simulink model "state_reg_mdl_2021a"  (R2021a)
settings: Solver=VariableStepAuto  StartTime=0.0  StopTime=20  RelTol=1e-3
values from neighbouring files (symbols this model uses):
  K = acker(A, B, p)    [state_reg.m]
  reg_type = 1    [state_reg.m]
  sat_off = 1    [state_reg.m]
  T = 1e-3    (= 0.001)    [state_reg.m]
  umax = 1    [state_reg.m]
libraries: simulink x1
settings Model: Creator=rapaja  LastModifiedBy=Predrag
settings SolverCC: AlgebraicLoopSolver=TrustRegion
settings RTWCC: DLArmComputeVersion=20.02.1
settings ConfigComp: CovBoundaryAbsTol=1.0e-5

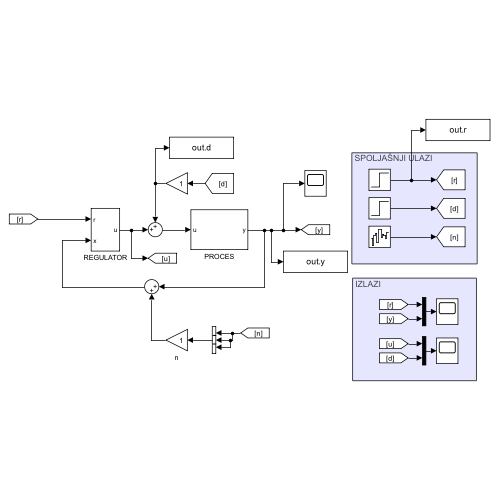
[thumbnail: Simulink's stored preview of the top-level diagram]
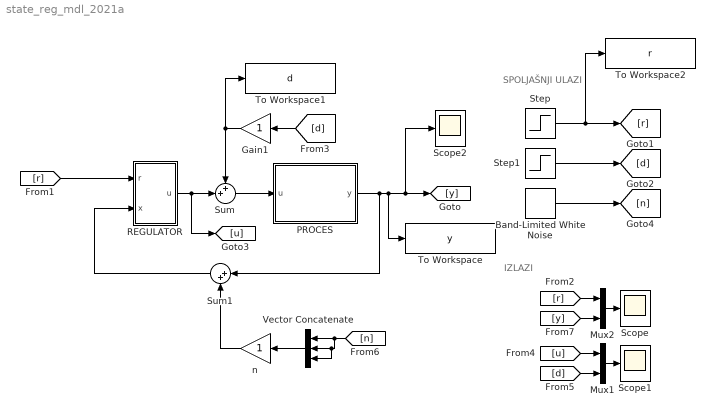
== system state_reg_mdl_2021a ==
  note: IZLAZI
  note: SPOLJAŠNJI ULAZI
  Band-Limited White Noise : simulink/Sources/Band-Limited White Noise  Cov=[0.00001]  Ts=T  seed=[23341]
  Gain1 : Gain
  Mux1 : Mux  Inputs=2
  Mux2 : Mux  Inputs=2
  PROCES : Subsystem
  REGULATOR : Subsystem
  Scope : Scope
  Scope1 : Scope
  Scope2 : Scope
  Step : Step  SampleTime=0
  Step1 : Step  Time=5  After=0  SampleTime=0
  Sum : Sum  Inputs=++|
  Sum1 : Sum  Inputs=|++
  To Workspace : ToWorkspace  VariableName=y  SampleTime=-1
  To Workspace1 : ToWorkspace  VariableName=d  SampleTime=-1
  To Workspace2 : ToWorkspace  VariableName=r  SampleTime=-1
  Vector Concatenate : Concatenate  NumInputs=3
  n : Gain
  wires:
  REGULATOR/1(u) -> [u], Sum/2
  [d] -> Gain1/1
  Band-Limited White Noise/1 -> [n]
  n/1 -> Sum1/2
  Gain1/1 -> To Workspace1/1, Sum/1
  Step1/1 -> [d]
  [r] -> Mux2/1
  [y] -> Mux2/2
  Mux2/1 -> Scope/1
  Mux1/1 -> Scope1/1
  [u] -> Mux1/1
  [d] -> Mux1/2
  PROCES/1(y) -> Sum1/1, To Workspace/1, Scope2/1, [y]
  [r] -> REGULATOR/1(r)
  Sum/1 -> PROCES/1(u)
  Sum1/1 -> REGULATOR/2(x)
  [n] -> Vector Concatenate/3, Vector Concatenate/2, Vector Concatenate/1
  Vector Concatenate/1 -> n/1
  Step/1 -> To Workspace2/1, [r]

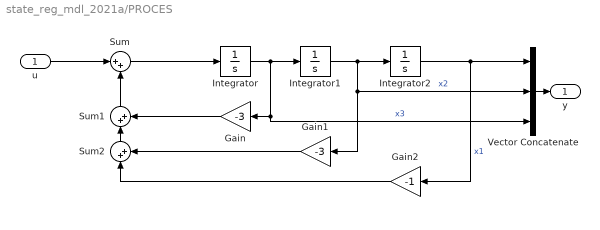
== system state_reg_mdl_2021a/PROCES ==
  u : Inport
  Gain : Gain  Gain=-3
  Gain1 : Gain  Gain=-3
  Gain2 : Gain  Gain=-1
  Integrator : Integrator
  Integrator1 : Integrator
  Integrator2 : Integrator
  Sum : Sum  Inputs=|++
  Sum1 : Sum  Inputs=|++
  Sum2 : Sum  Inputs=|++
  Vector Concatenate : Concatenate  NumInputs=3
  y : Outport
  wires:
  Vector Concatenate/1 -> y/1
  Integrator2/1 -> Gain2/1, Vector Concatenate/1  "x1"
  Integrator1/1 -> Vector Concatenate/2, Gain1/1, Integrator2/1  "x2"
  Integrator/1 -> Vector Concatenate/3, Gain/1, Integrator1/1  "x3"
  u/1 -> Sum/1
  Sum/1 -> Integrator/1
  Gain/1 -> Sum1/2
  Sum1/1 -> Sum/2
  Sum2/1 -> Sum1/1
  Gain1/1 -> Sum2/2
  Gain2/1 -> Sum2/1

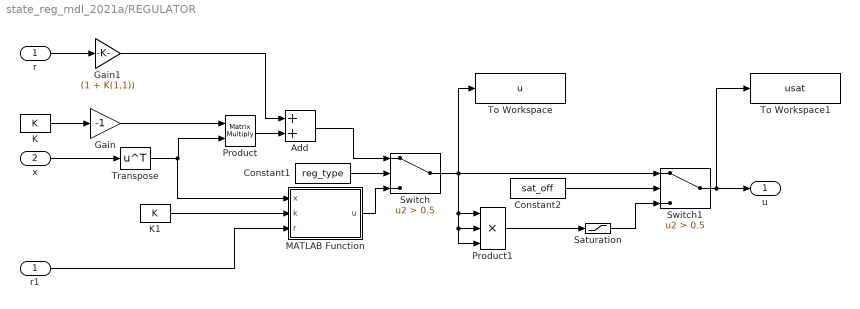
== system state_reg_mdl_2021a/REGULATOR ==
  r : Inport
  x : Inport  Port=2
  Add : Sum
  Constant1 : Constant  Value=reg_type
  Constant2 : Constant  Value=sat_off
  Gain : Gain  Gain=-1
  Gain1 : Gain  Gain=(1 + K(1,1))
  K : Constant  Value=K  VectorParams1D=off
  K1 : Constant  Value=K  VectorParams1D=off
  MATLAB Function : MATLAB Function  TreatAsAtomicUnit=on  SystemSampleTime=T
  Product : Product  Multiplication=Matrix(*)
  Product1 : Product  Inputs=3
  Saturation : Saturate  UpperLimit=umax  LowerLimit=-umax
  Switch : Switch  Criteria=u2 > Threshold  Threshold=0.5
  Switch1 : Switch  Criteria=u2 > Threshold  Threshold=0.5
  To Workspace : ToWorkspace  VariableName=u  SampleTime=-1
  To Workspace1 : ToWorkspace  VariableName=usat  SampleTime=-1
  Transpose : Math  Operator=transpose  SaturateOnIntegerOverflow=on
  r1 : InportShadow
  u : Outport
  wires:
  K/1 -> Gain/1
  r/1 -> Gain1/1
  Gain1/1 -> Add/1
  Product/1 -> Add/2
  Switch/1 -> Switch1/1, Product1/3, Product1/2, Product1/1, To Workspace/1
  MATLAB Function/1(u) -> Switch/3
  Add/1 -> Switch/1
  Constant1/1 -> Switch/2
  Gain/1 -> Product/1
  K1/1 -> MATLAB Function/2(k)
  Transpose/1 -> MATLAB Function/1(x), Product/2
  x/1 -> Transpose/1
  r1/1 -> MATLAB Function/3(r)
  Switch1/1 -> To Workspace1/1, u/1
  Saturation/1 -> Switch1/3
  Constant2/1 -> Switch1/2
  Product1/1 -> Saturation/1

== matlab function state_reg_mdl_2021a/REGULATOR/MATLAB Function ==
  data: x input; u output; k input; r input
function u = fcn(x, k, r)

u = -k*x + (1 + k(1, 1)) * r;
